simulink model "old_model"  (R2020b)
settings: Solver=VariableStepAuto  StartTime=0.0  StopTime=100  RelTol=1e-3
undefined symbols (not defined in the file or in its folder): Ion, Lithium
libraries: powerlib x12, electricdrivelib x4
settings Model: SimulationMode=accelerator  Creator=amrat  LastModifiedBy=amrat

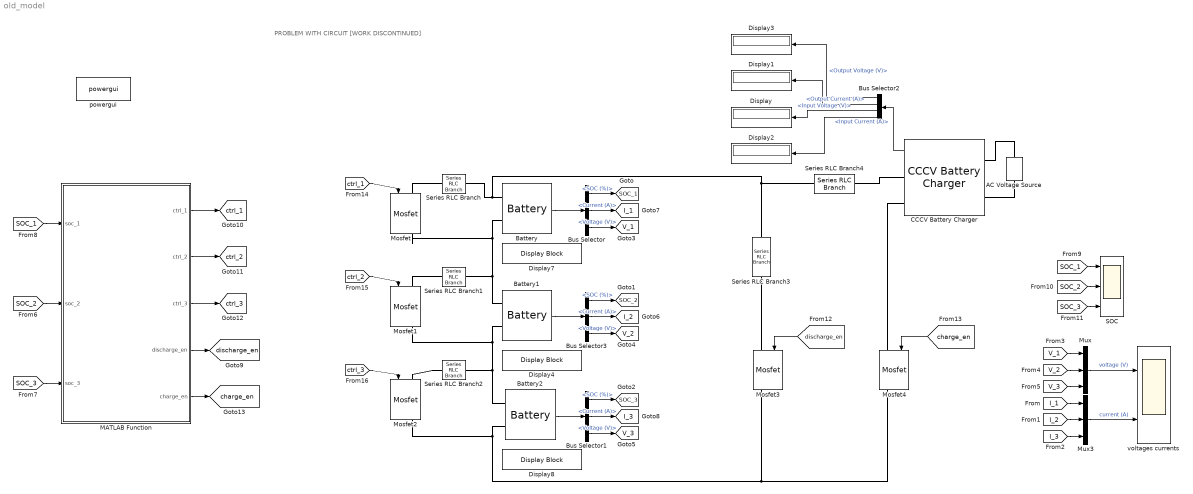
== system old_model ==
  note: PROBLEM WITH CIRCUIT [WORK DISCONTINUED]
  AC Voltage Source : powerlib/Electrical Sources/AC Voltage Source  Amplitude=325  Phase=0  Frequency=60  SampleTime=0  Measurements=None  BusType=swing  Pref=10e3  Qref=0  Qmin=-inf  Qmax=+inf
  Battery : electricdrivelib/Extra Sources/Battery  BatType=Lithium-Ion  ShowTempParam=off  ThermalPreset=no  ShowAgeParam=off  NomV=3.7  NomQ=1.5  SOC=10  Batt_Tr=0.5  PresetModel=off  MaxQ=1.5  MinV=2.775  FullV=4.3068  Dis_rate=1.25117  R=2.195667  Normal_OP=1.3565  expZone="[3.9974    0.073696]"  current=[6.5 13 32.5]  Units=Time  Tci=20  NomT=20  T2=-30  MaxQ2=4.8  FullV2=7.1  Normal_OP2=5.655  expZone2="[6.58           1]"  Rca=0.6  ti=2000  Dp=0  Neq0=0  Tsim=1e6  Ta1=25  Qeol=5.4*0.9  Reol=0.013333*1.2  Char_age=[2.3478, 3]  Dis_age=[2.3478, 10]  N1=1500  N2=10500  N3=1000  N4=1400  Ta2=45  N5=950
  Battery1 : electricdrivelib/Extra Sources/Battery  BatType=Lithium-Ion  ShowTempParam=off  ThermalPreset=no  ShowAgeParam=off  NomV=3.7  NomQ=1.5  SOC=1  Batt_Tr=0.5  PresetModel=on  MaxQ=1.5  MinV=2.775  FullV=4.3068  Dis_rate=0.65217  R=0.024667  Normal_OP=1.3565  expZone="[3.9974    0.073696]"  current=[6.5 13 32.5]  Units=Time  Tci=20  NomT=20  T2=-30  MaxQ2=4.8  FullV2=7.1  Normal_OP2=5.655  expZone2="[6.58           1]"  Rca=0.6  ti=2000  Dp=0  Neq0=0  Tsim=1e6  Ta1=25  Qeol=5.4*0.9  Reol=0.013333*1.2  Char_age=[2.3478, 3]  Dis_age=[2.3478, 10]  N1=1500  N2=10500  N3=1000  N4=1400  Ta2=45  N5=950
  Battery2 : electricdrivelib/Extra Sources/Battery  BatType=Lithium-Ion  ShowTempParam=off  ThermalPreset=no  ShowAgeParam=off  NomV=3.7  NomQ=1.5  SOC=65  Batt_Tr=0.5  PresetModel=off  MaxQ=1.5  MinV=2.775  FullV=4.3068  Dis_rate=0.64217  R=0.014667  Normal_OP=1.3565  expZone="[3.9974    0.073696]"  current=[6.5 13 32.5]  Units=Time  Tci=20  NomT=20  T2=-30  MaxQ2=4.8  FullV2=7.1  Normal_OP2=5.655  expZone2="[6.58           1]"  Rca=0.6  ti=2000  Dp=0  Neq0=0  Tsim=1e6  Ta1=25  Qeol=5.4*0.9  Reol=0.013333*1.2  Char_age=[2.3478, 3]  Dis_age=[2.3478, 10]  N1=1500  N2=10500  N3=1000  N4=1400  Ta2=45  N5=950
  Bus Selector : BusSelector  OutputSignals=SOC (%),Current (A),Voltage (V)
  Bus Selector1 : BusSelector  OutputSignals=SOC (%),Current (A),Voltage (V)
  Bus Selector2 : BusSelector  OutputSignals=Output Voltage (V),Output Current (A),Input Voltage (V),Input Current (A)
  Bus Selector3 : BusSelector  OutputSignals=SOC (%),Current (A),Voltage (V)
  CCCV Battery Charger : electricdrivelib/Extra Sources/CCCV Battery Charger  Preset=Custom specifications  P_nom=1500  s_type=1-phase AC  n_connect=off  eff_volt=230  in_freq=60  in_I_ripple=10  in_I_freq=1000  EFF_en=on  EFF_val=[0.627 0.803 0.855 0.871 0.872 0.864]  EFF_fu=[0.063 0.177 0.293 0.483 0.674 0.914]  THD_en=on  I_THD_val=[0.327 0.394 0.394 0.351 0.289 0.265]  I_THD_fu=[0.056 0.136 0.194 0.303 0.555 0.916]  H_DIST_rt=[0.199 1.297 0.328 0.029 0.416 0.200]  H_DIST_fr=[3 5 7 9 11 13]  PF_en=on  PF_val=[0.316 0.532 0.662 0.731 0.780 0.792]  PF_fu=[0.067 0.230 0.445 0.625 0.794 0.919]  Out_mode=Constant Current - Constant Voltage (CCCV)  DynInT=off  I_cst=1.5  V_cst=4.2  ABS_en=off  V_abs=142  ABS_end=Time based  ABS_time=3600  ABS_i=40  ripple=0.5  swF=1000  overshoot=1  stable_t=2  VoltComp=off  V_comp=-0.18  nom_temp=20
      settings: SourceProductBaseCode=PS
  Display{,1..3} (4 alike) : Display
  Display4 : DisplayBlock  LabelPosition=Hide  Format=Custom  Transparency=1  FormatString=%0.2f
  Display7 : DisplayBlock  LabelPosition=Hide  Format=Custom  Transparency=1  FormatString=%0.2f
  Display8 : DisplayBlock  LabelPosition=Hide  Format=Custom  Transparency=1  FormatString=%0.2f
  MATLAB Function : MATLAB Function  TreatAsAtomicUnit=on
  Mosfet{,1..4} (5 alike) : powerlib/Power Electronics/Mosfet  Ron=0.1  Lon=0  Rd=0.01  Vfd=0  IC=0  Rs=1e5  Cs=inf  Measurements=on
  Mux : Mux  Inputs=3
  Mux3 : Mux  Inputs=3
  SOC : Scope  NumInputPorts=3
  Series RLC Branch : powerlib/Elements/Series RLC Branch  LConnTagsString=__new0  RConnTagsString=__new0  BranchType=R  Resistance=3  Inductance=1e-3  SetiL0=off  InitialCurrent=0  Capacitance=1e-6  Setx0=off  InitialVoltage=0  Measurements=None
  Series RLC Branch1 : powerlib/Elements/Series RLC Branch  LConnTagsString=__new0  RConnTagsString=__new0  BranchType=R  Resistance=3  Inductance=1e-3  SetiL0=off  InitialCurrent=0  Capacitance=1e-6  Setx0=off  InitialVoltage=0  Measurements=None
  Series RLC Branch2 : powerlib/Elements/Series RLC Branch  LConnTagsString=__new0  RConnTagsString=__new0  BranchType=R  Resistance=3  Inductance=1e-3  SetiL0=off  InitialCurrent=0  Capacitance=1e-6  Setx0=off  InitialVoltage=0  Measurements=None
  Series RLC Branch3 : powerlib/Elements/Series RLC Branch  LConnTagsString=__new0  RConnTagsString=__new0  BranchType=R  Resistance=4  Inductance=1e-3  SetiL0=off  InitialCurrent=0  Capacitance=1e-6  Setx0=off  InitialVoltage=0  Measurements=None
  Series RLC Branch4 : powerlib/Elements/Series RLC Branch  LConnTagsString=__new0  RConnTagsString=__new0  BranchType=R  Resistance=4  Inductance=1e-3  SetiL0=off  InitialCurrent=0  Capacitance=1e-6  Setx0=off  InitialVoltage=0  Measurements=None
  powergui : powerlib/powergui  Priority=1  SimulationMode=Continuous  SampleTime=50e-6  frequency=60  Iterations=50  frequencyindice=0  Pbase=100e6  ErrMax=1e-4  UnitsV=kV  UnitsW=MW  buscounter=0  FunctionMessages=off  echomessages=off  EnableUseOfTLC=off  CurrentSourceSwitches=off  DisableSnubberDevices=off  DisableRonSwitches=off  DisableVfSwitches=off  DisplayEquations=off  AutomaticDiscreteSolvers=off  SolverType=Tustin/Backward Euler (TBE)  Interpol=off  ExternalGateDelay=off  methode=off  Ts=100  x0status=blocks  SPID=on  SwTol=0  HookPort=off  NonlinearTolerance=1e-4  nMaxIteration=100  ContinueOnMaxIteration=off  RestoreLinks=warning  ResistiveCurrentMeasurement=off  Frange=[0:2:500]  Ylog=off  Xlog=on  ShowGrid=off  save=off  variable=ZData  structure=0  ZoomFFT=off  StartTime=0.0  cycles=1  DisplayStyle=1  fundamental=60  FreqAxis=off  MaxFrequency=1000  frequencyindicesteady=1  RmsSteady=1  display=off
  voltages currents : Scope  NumInputPorts=2
  tag scope: I_1=global, I_2=global, I_3=global, SOC_1=global, SOC_2=global, SOC_3=global, V_1=global, V_2=global, V_3=global, charge_en=global, ctrl_1=global, ctrl_2=global, ctrl_3=global, discharge_en=global
  wires:
  Battery/1 -> Bus Selector/1
  Battery2/1 -> Bus Selector1/1
  Bus Selector/2 -> [I_1]  "<Current (A)>"
  Battery1/1 -> Bus Selector3/1
  Bus Selector3/1 -> [SOC_2]  "<SOC (%)>"
  Bus Selector1/1 -> [SOC_3]  "<SOC (%)>"
  Bus Selector3/3 -> [V_2]  "<Voltage (V)>"
  Bus Selector/3 -> [V_1]  "<Voltage (V)>"
  Bus Selector3/2 -> [I_2]  "<Current (A)>"
  Bus Selector1/3 -> [V_3]  "<Voltage (V)>"
  Bus Selector1/2 -> [I_3]  "<Current (A)>"
  Mux3/1 -> voltages currents/2  "current (A)"
  Mux/1 -> voltages currents/1  "voltage (V)"
  [I_1] -> Mux3/1
  [I_2] -> Mux3/2
  [I_3] -> Mux3/3
  [V_1] -> Mux/1
  [V_2] -> Mux/2
  [V_3] -> Mux/3
  [SOC_2] -> SOC/2
  [SOC_3] -> SOC/3
  [SOC_1] -> SOC/1
  Bus Selector/1 -> [SOC_1]  "<SOC (%)>"
  [discharge_en] -> Mosfet3/1
  [charge_en] -> Mosfet4/1
  MATLAB Function/1(ctrl_1) -> [ctrl_1]
  MATLAB Function/2(ctrl_2) -> [ctrl_2]
  MATLAB Function/3(ctrl_3) -> [ctrl_3]
  MATLAB Function/4(discharge_en) -> [discharge_en]
  MATLAB Function/5(charge_en) -> [charge_en]
  [SOC_3] -> MATLAB Function/3(soc_3)
  [SOC_2] -> MATLAB Function/2(soc_2)
  [SOC_1] -> MATLAB Function/1(soc_1)
  [ctrl_1] -> Mosfet/1
  [ctrl_2] -> Mosfet1/1
  [ctrl_3] -> Mosfet2/1
  CCCV Battery Charger/1 -> Bus Selector2/1
  Bus Selector2/1 -> Display3/1  "<Output Voltage (V)>"
  Bus Selector2/2 -> Display1/1  "<Output Current (A)>"
  Bus Selector2/3 -> Display/1  "<Input Voltage (V)>"
  Bus Selector2/4 -> Display2/1  "<Input Current (A)>"
  connections:
  Battery/LConn2 -- Mosfet/RConn1 -- Battery1/LConn1 -- Series RLC Branch1/RConn1
  Battery1/LConn2 -- Mosfet1/RConn1 -- Series RLC Branch2/RConn1 -- Battery2/LConn1
  Mosfet/LConn1 -- Series RLC Branch/LConn1
  Mosfet1/LConn1 -- Series RLC Branch1/LConn1
  Series RLC Branch2/LConn1 -- Mosfet2/LConn1
  Mosfet2/RConn1 -- Mosfet3/RConn1 -- Mosfet4/RConn1 -- Battery2/LConn2
  Mosfet3/LConn1 -- Series RLC Branch3/RConn1
  Series RLC Branch/RConn1 -- Series RLC Branch4/RConn1 -- Series RLC Branch3/LConn1 -- Battery/LConn1
  CCCV Battery Charger/LConn2 -- AC Voltage Source/LConn1
  CCCV Battery Charger/LConn1 -- AC Voltage Source/RConn1
  Series RLC Branch4/LConn1 -- CCCV Battery Charger/RConn1
  Mosfet4/LConn1 -- CCCV Battery Charger/RConn2

== matlab function old_model/MATLAB Function ==
  data: soc_1 input; ctrl_1 output; soc_2 input; soc_3 input; ctrl_2 output; ctrl_3 output; discharge_en output; charge_en output
function [ctrl_1,ctrl_2,ctrl_3,discharge_en,charge_en] = bal_algorithm(soc_1,soc_2,soc_3)
discharge_en = 2;
charge_en = 0;
end
